simulink model "switch_SCV"  (R2024a)
settings: Solver=VariableStepAuto  StartTime=0.0  StopTime=0.2  RelTol=1e-3
libraries: spsThreePhaseBreakerLib x3, spsUniversalBridgeLib x2, spsPower3phInstantaneousLib x1, spsSeriesRLCBranchLib x1, spsSynchronousMachinepuFundamentalLib x1, spsThreePhaseParallelRLCLoadLib x1, spsThreePhaseSeriesRLCLoadLib x1, spsThreePhaseVIMeasurementLib x1, spsThreePhaseSourceLib x1, sps_lib x1
settings Model: Creator=User  LastModifiedBy=User

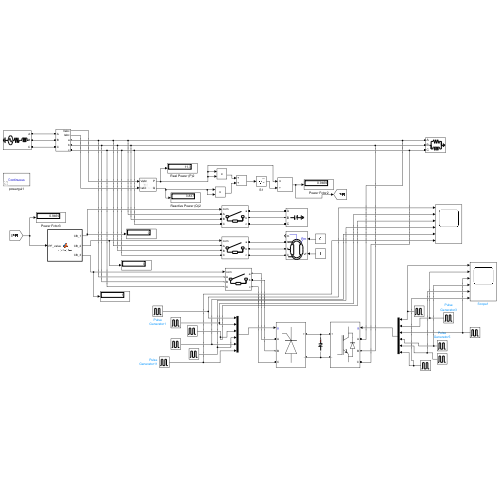
[thumbnail: Simulink's stored preview of the top-level diagram]
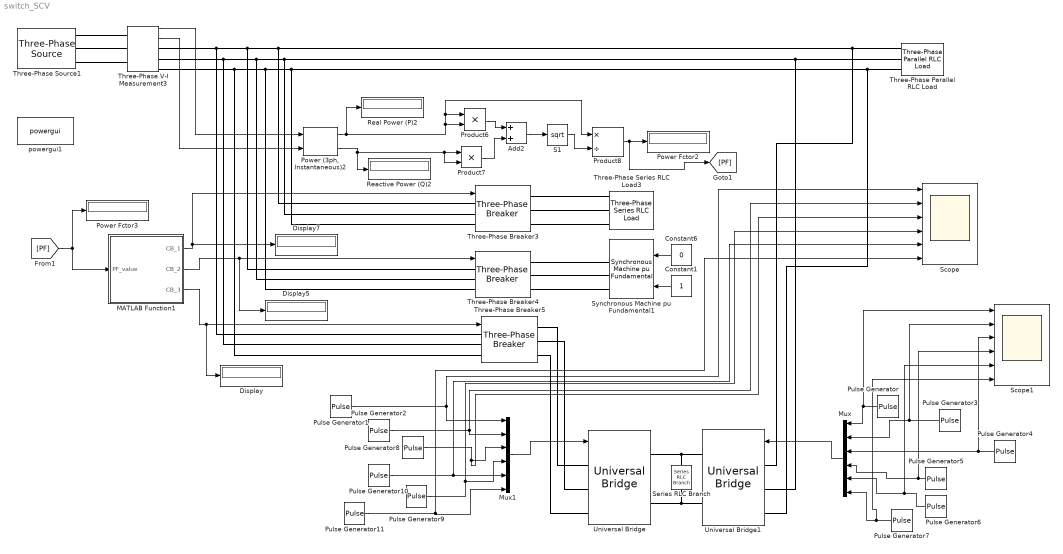
== system switch_SCV ==
  Add2 : Sum
  Constant1 : Constant
  Constant6 : Constant  Value=0
  Display : Display
  Display5 : Display
  Display7 : Display
  MATLAB Function1 : MATLAB Function  TreatAsAtomicUnit=on
  Mux : Mux  Inputs=6
  Mux1 : Mux  Inputs=6
  "Power (3ph, Instantaneous)2" : spsPower3phInstantaneousLib/Power (3ph, Instantaneous)
  Power Fctor2 : Display
  Power Fctor3 : Display
  Product6 : Product
  Product7 : Product
  Product8 : Product  Inputs=*/
  Pulse Generator : DiscretePulseGenerator  PulseType=Time based  Period=1/50  PulseWidth=50  PhaseDelay=0.02/6
  Pulse Generator1 : DiscretePulseGenerator  PulseType=Time based  Period=1/50  PulseWidth=6.667e-3
  Pulse Generator10 : DiscretePulseGenerator  PulseType=Time based  Period=1/50  PulseWidth=6.667e-3  PhaseDelay=240
  Pulse Generator11 : DiscretePulseGenerator  PulseType=Time based  Period=1/50  PulseWidth=6.667e-3  PhaseDelay=300
  Pulse Generator2 : DiscretePulseGenerator  PulseType=Time based  Period=1/50  PulseWidth=6.667e-3  PhaseDelay=60
  Pulse Generator3 : DiscretePulseGenerator  PulseType=Time based  Period=0.02  PulseWidth=50  PhaseDelay=2*(0.02/6)
  Pulse Generator4 : DiscretePulseGenerator  PulseType=Time based  Period=0.02  PulseWidth=50  PhaseDelay=3*(0.02/6)
  Pulse Generator5 : DiscretePulseGenerator  PulseType=Time based  Period=0.02  PulseWidth=50  PhaseDelay=4*(0.02/6)
  Pulse Generator6 : DiscretePulseGenerator  PulseType=Time based  Period=0.02  PulseWidth=50  PhaseDelay=5*(0.02/6)
  Pulse Generator7 : DiscretePulseGenerator  PulseType=Time based  Period=0.020  PulseWidth=50  PhaseDelay=6*(0.020/6)
  Pulse Generator8 : DiscretePulseGenerator  PulseType=Time based  Period=1/50  PulseWidth=6.667e-3  PhaseDelay=120
  Pulse Generator9 : DiscretePulseGenerator  PulseType=Time based  Period=1/50  PulseWidth=6.667e-3  PhaseDelay=180
  Reactive Power (Q)2 : Display
  Real Power (P)2 : Display
  S1 : Sqrt
  Scope : Scope  NumInputPorts=6
  Scope1 : Scope  NumInputPorts=6
  Series RLC Branch : spsSeriesRLCBranchLib/Series RLC Branch  LConnTagsString=__new0  RConnTagsString=__new0  BranchType=C  Resistance=1  Inductance=1e-3  SetiL0=off  InitialCurrent=0  Capacitance=1e-6  Setx0=off  InitialVoltage=0  Measurements=None
  Synchronous Machine pu Fundamental1 : spsSynchronousMachinepuFundamentalLib/Synchronous Machine pu Fundamental  PresetModel=No  MechanicalLoad=Mechanical power Pm  ShowDetailedParameters=on  RotorType=Salient-pole  Units=per unit fundamental parameters  MeasurementBus=on  NominalParameters="[ 4e3  400   50]"  Stator="[ 2.85E-03  0.114  1.19  0.36 ]"  Field="[ 5.79E-04  0.114]"  Dampers2=[0.0652, 0.5134, 0.0287, 0.2553, 7.765e-3, 0.9167 ]  Dampers1="[ 1.17E-02  0.182  1.97E-02  0.384 ]"  Mechanical=[ 3.7 0 20]  PolePairs=20  InitialConditions="[ 0  0  0  0  0  0  0  0  1 ]"  SetSaturation=off  Saturation=[0.6404,0.7127,0.8441,0.9214,0.9956,1.082,1.19,1.316,1.457;0.7,0.7698,0.8872,0.9466,0.9969,1.046,1.1,1.151,1.201]  LoadFlowParameters=[1,0,0,0,0]  TsPowergui=0  TsBlock=-1  IterativeModel=Trapezoidal non iterative  IterativeDiscreteModel=Trapezoidal non iterative  BusType=PV  Pref=0  Qref=0  Qmin=-inf  Qmax=inf  PLF=0  QLF=0
      settings: LibrarySourceBlock=|
      | sps_lib/Electrical Machines/Synchronous Machine
      | pu Fundamental
  Three-Phase Parallel RLC Load : spsThreePhaseParallelRLCLoadLib/Three-Phase Parallel RLC Load  LConnTagsString=A|B|C  Configuration=Y (grounded)  NominalVoltage=400  Vabc=[1e3 1e3 1e3]  Vabcp=[1e3 1e3 1e3]  NominalFrequency=50  UnbalancedPower=off  ActivePower=5e3  InductivePower=7000  CapacitivePower=0  Pabc=[10e3 9e3 11e3]  QLabc=[100 90 110]  QCabc=[100 90 110]  Pabcp=[10e3 9e3 11e3]  QLabcp=[100 90 110]  QCabcp=[100 90 110]  Measurements=None  LoadType=constant PQ
  Three-Phase Series RLC Load3 : spsThreePhaseSeriesRLCLoadLib/Three-Phase Series RLC Load  LConnTagsString=A|B|C  Configuration=Y (grounded)  NominalVoltage=400  Vabc=[1e3 1e3 1e3]  Vabcp=[1e3 1e3 1e3]  NominalFrequency=50  UnbalancedPower=off  ActivePower=0  InductivePower=0  CapacitivePower=1.5e3  Pabc=[10e3 9e3 11e3]  QLabc=[100 90 110]  QCabc=[100 90 110]  Pabcp=[10e3 9e3 11e3]  QLabcp=[100 90 110]  QCabcp=[100 90 110]  Measurements=None  LoadType=constant Z
  Three-Phase V-I Measurement3 : spsThreePhaseVIMeasurementLib/Three-Phase V-I Measurement  VoltageMeasurement=phase-to-ground  SetLabelV=off  LabelV=Vabc  Vpu=off  VpuLL=off  CurrentMeasurement=yes  SetLabelI=off  LabelI=Iabc  Ipu=off  Pbase=100e6  Vbase=500e3  OutputType=Complex  PhasorSimulation=off  PSBequivalent=0
  Three-Phase Breaker3 : spsThreePhaseBreakerLib/Three-Phase Breaker  InitialState=open  SwitchA=on  SwitchB=on  SwitchC=on  SwitchTimes="[1/60  5/60]"  External=on  BreakerResistance=0.01  SnubberResistance=1e6  SnubberCapacitance=inf  Measurements=None
  Three-Phase Breaker4 : spsThreePhaseBreakerLib/Three-Phase Breaker  InitialState=open  SwitchA=on  SwitchB=on  SwitchC=on  SwitchTimes="[1/60  5/60]"  External=on  BreakerResistance=0.01  SnubberResistance=1e6  SnubberCapacitance=inf  Measurements=None
  Three-Phase Breaker5 : spsThreePhaseBreakerLib/Three-Phase Breaker  InitialState=open  SwitchA=on  SwitchB=on  SwitchC=on  SwitchTimes="[1/60  5/60]"  External=on  BreakerResistance=0.01  SnubberResistance=1e6  SnubberCapacitance=inf  Measurements=None
  Three-Phase Source1 : spsThreePhaseSourceLib/Three-Phase Source  InternalConnection=Yg  VoltagePhases=off  Voltage=400  PhaseAngle=0  Voltage_phases=[25e3 25e3 25e3]/sqrt(3)  PhaseAngles_phases=[0 -120 +120]  Frequency=50  NonIdealSource=on  SpecifyImpedance=off  Resistance=0.8929  Inductance=16.58e-3  ShortCircuitLevel=1200  BaseVoltage=400  XRratio=7  BusType=swing  Pref=10e3  Qref=0  Prefabc=[10e3, 10e3, 10e3]  Qrefabc=[0, 0, 0]  Qmin=-inf  Qmax=inf
  Universal Bridge : spsUniversalBridgeLib/Universal Bridge  Arms=3  SnubberResistance=1e5  SnubberCapacitance=inf  Device=Thyristors  Ron=1e-3  Lon=0  ForwardVoltages="[  0  0  ]"  ForwardVoltage=0  GTOparameters=[ 10e-6 , 20e-6 ]  IGBTparameters=[ 1e-6 , 2e-6 ]  Measurements=None  Measurements_2=None  converterType=Rectifier
  Universal Bridge1 : spsUniversalBridgeLib/Universal Bridge  Arms=3  SnubberResistance=1e5  SnubberCapacitance=inf  Device=IGBT / Diodes  Ron=1e-3  Lon=0  ForwardVoltages="[  400  400  ]"  ForwardVoltage=0  GTOparameters=[ 10e-6 , 20e-6 ]  IGBTparameters=[ 1e-6 , 2e-6 ]  Measurements=None  Measurements_2=None  converterType=Rectifier
  powergui1 : sps_lib/powergui  Priority=1  SimulationMode=Continuous  SampleTime=50e-6  frequency=60  Iterations=50  frequencyindice=50  Pbase=100e6  ErrMax=1e-4  UnitsV=kV  UnitsW=MW  buscounter=0  FunctionMessages=off  echomessages=off  EnableUseOfTLC=off  CurrentSourceSwitches=off  DisableSnubberDevices=off  DisableRonSwitches=off  DisableVfSwitches=off  DisplayEquations=off  AutomaticDiscreteSolvers=off  SolverType=Tustin/Backward Euler (TBE)  Interpol=off  ExternalGateDelay=off  methode=off  Ts=100  x0status=blocks  SPID=on  SwTol=0  HookPort=off  NonlinearTolerance=1e-4  nMaxIteration=100  ContinueOnMaxIteration=off  RestoreLinks=warning  ResistiveCurrentMeasurement=off  Frange=[0:2:500]  Ylog=off  Xlog=on  ShowGrid=off  save=off  variable=ZData  structure=0  ZoomFFT=off  StartTime=0.0  cycles=1  DisplayStyle=1  fundamental=60  FreqAxis=off  MaxFrequency=1000  frequencyindicesteady=1  RmsSteady=1  display=off
  wires:
  MATLAB Function1/1(CB_1) -> Display7/1, Three-Phase Breaker3/1
  "Power (3ph, Instantaneous)2"/2 -> Reactive Power (Q)2/1, Product7/2, Product7/1
  [PF] -> Power Fctor3/1, MATLAB Function1/1(PF_value)
  Add2/1 -> S1/1
  Three-Phase V-I Measurement3/1 -> "Power (3ph, Instantaneous)2"/1
  "Power (3ph, Instantaneous)2"/1 -> Real Power (P)2/1, Product8/1, Product6/1, Product6/2
  Three-Phase V-I Measurement3/2 -> "Power (3ph, Instantaneous)2"/2
  Product8/1 -> [PF], Power Fctor2/1
  Product6/1 -> Add2/1
  Product7/1 -> Add2/2
  S1/1 -> Product8/2
  Constant6/1 -> Synchronous Machine pu Fundamental1/1
  Constant1/1 -> Synchronous Machine pu Fundamental1/2
  Mux1/1 -> Universal Bridge/1
  Pulse Generator7/1 -> Scope1/6, Mux/6
  Mux/1 -> Universal Bridge1/1
  Pulse Generator6/1 -> Mux/5, Scope1/5
  Pulse Generator5/1 -> Mux/4, Scope1/4
  Pulse Generator4/1 -> Scope1/3, Mux/3
  Pulse Generator/1 -> Scope1/1, Mux/1
  Pulse Generator3/1 -> Scope1/2, Mux/2
  Pulse Generator9/1 -> Scope/4, Mux1/4
  Pulse Generator11/1 -> Mux1/6, Scope/6
  Pulse Generator2/1 -> Mux1/2, Scope/2
  Pulse Generator1/1 -> Mux1/1, Scope/1
  Pulse Generator8/1 -> Scope/3, Mux1/3
  Pulse Generator10/1 -> Scope/5, Mux1/5
  MATLAB Function1/2(CB_2) -> Display5/1, Three-Phase Breaker4/1
  MATLAB Function1/3(CB_3) -> Display/1, Three-Phase Breaker5/1
  connections:
  Three-Phase V-I Measurement3/RConn1 -- Three-Phase Breaker5/LConn1 -- Universal Bridge1/LConn1 -- Three-Phase Parallel RLC Load/LConn1 -- Three-Phase Breaker3/LConn1 -- Three-Phase Breaker4/LConn1
  Three-Phase V-I Measurement3/RConn3 -- Three-Phase Breaker5/LConn3 -- Three-Phase Breaker4/LConn3 -- Universal Bridge1/LConn3 -- Three-Phase Parallel RLC Load/LConn3 -- Three-Phase Breaker3/LConn3
  Three-Phase V-I Measurement3/RConn2 -- Three-Phase Breaker5/LConn2 -- Three-Phase Parallel RLC Load/LConn2 -- Universal Bridge1/LConn2 -- Three-Phase Breaker3/LConn2 -- Three-Phase Breaker4/LConn2
  Three-Phase Source1/RConn2 -- Three-Phase V-I Measurement3/LConn2
  Three-Phase Breaker3/RConn3 -- Three-Phase Series RLC Load3/LConn3
  Three-Phase Series RLC Load3/LConn1 -- Three-Phase Breaker3/RConn1
  Three-Phase Source1/RConn3 -- Three-Phase V-I Measurement3/LConn3
  Three-Phase Breaker3/RConn2 -- Three-Phase Series RLC Load3/LConn2
  Three-Phase Source1/RConn1 -- Three-Phase V-I Measurement3/LConn1
  Synchronous Machine pu Fundamental1/RConn1 -- Three-Phase Breaker4/RConn1
  Synchronous Machine pu Fundamental1/RConn2 -- Three-Phase Breaker4/RConn2
  Synchronous Machine pu Fundamental1/RConn3 -- Three-Phase Breaker4/RConn3
  Three-Phase Breaker5/RConn3 -- Universal Bridge/LConn3
  Three-Phase Breaker5/RConn1 -- Universal Bridge/LConn1
  Three-Phase Breaker5/RConn2 -- Universal Bridge/LConn2
  Universal Bridge/RConn1 -- Universal Bridge1/RConn1 -- Series RLC Branch/LConn1
  Universal Bridge/RConn2 -- Universal Bridge1/RConn2 -- Series RLC Branch/RConn1

== matlab function switch_SCV/MATLAB Function1 ==
  data: PF_value input; CB_1 output; CB_2 output; CB_3 output
function [CB_1,CB_2,CB_3] = controller(PF_value)

if (PF_value<=0.60)
    CB_1=1;
    CB_2=0;
    CB_3=0;

elseif (PF_value<=0.75)
    CB_1=0;
    CB_2=1;
    CB_3=0;

elseif (PF_value<=0.85)
    CB_1=0;
    CB_2=0;
    CB_3=1;
else 
    CB_1=0;
    CB_2=0;
    CB_3=1;
end

end
